simulink library "lut_ram_vhdl"  (R2013b)
settings: Solver=ode45  StartTime=0.0  StopTime=10.0  RelTol=1e-3
libraries: xbsIndex_r4 x27
settings Model: Creator=eyonfen  LastModifiedBy=Administrator

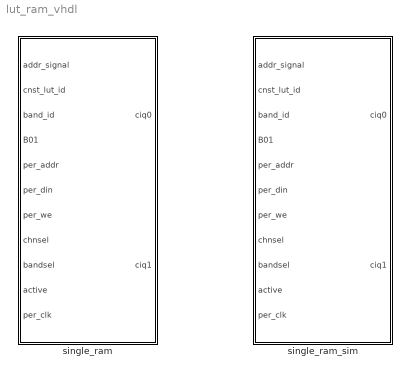
== system lut_ram_vhdl ==
  single_ram : Subsystem
  single_ram_sim : Subsystem

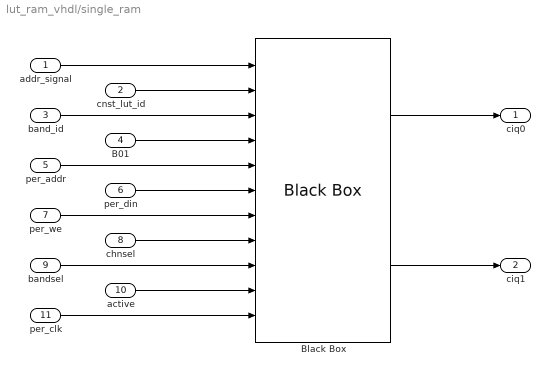
== system lut_ram_vhdl/single_ram ==
  addr_signal : Inport
  cnst_lut_id : Inport  Port=2
  band_id : Inport  Port=3
  B01 : Inport  Port=4
  per_addr : Inport  Port=5
  per_din : Inport  Port=6
  per_we : Inport  Port=7
  chnsel : Inport  Port=8
  bandsel : Inport  Port=9
  active : Inport  Port=10
  per_clk : Inport  Port=11
  Black Box : xbsIndex_r4/Black Box  init_code=dim2lut_config  sim_method=Inactive  verbose=off  block_type=blackbox2
  ciq0 : Outport
  ciq1 : Outport  Port=2
  wires:
  Black Box/1 -> ciq0/1
  Black Box/2 -> ciq1/1
  addr_signal/1 -> Black Box/1
  cnst_lut_id/1 -> Black Box/2
  band_id/1 -> Black Box/3
  B01/1 -> Black Box/4
  per_addr/1 -> Black Box/5
  per_din/1 -> Black Box/6
  per_we/1 -> Black Box/7
  chnsel/1 -> Black Box/8
  bandsel/1 -> Black Box/9
  active/1 -> Black Box/10
  per_clk/1 -> Black Box/11

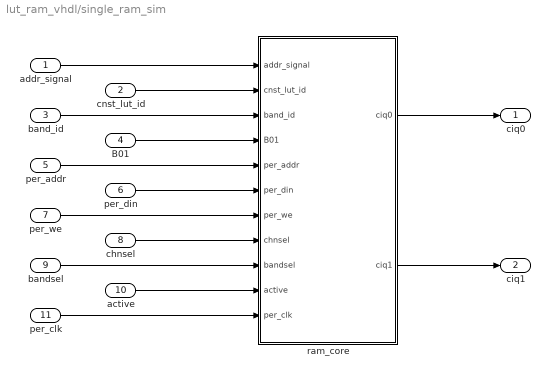
== system lut_ram_vhdl/single_ram_sim ==
  addr_signal : Inport
  cnst_lut_id : Inport  Port=2
  band_id : Inport  Port=3
  B01 : Inport  Port=4
  per_addr : Inport  Port=5
  per_din : Inport  Port=6
  per_we : Inport  Port=7
  chnsel : Inport  Port=8
  bandsel : Inport  Port=9
  active : Inport  Port=10
  per_clk : Inport  Port=11
  ram_core : Subsystem
  ciq0 : Outport
  ciq1 : Outport  Port=2
  wires:
  ram_core/1(ciq0) -> ciq0/1
  ram_core/2(ciq1) -> ciq1/1
  addr_signal/1 -> ram_core/1(addr_signal)
  cnst_lut_id/1 -> ram_core/2(cnst_lut_id)
  band_id/1 -> ram_core/3(band_id)
  B01/1 -> ram_core/4(B01)
  per_addr/1 -> ram_core/5(per_addr)
  per_din/1 -> ram_core/6(per_din)
  per_we/1 -> ram_core/7(per_we)
  chnsel/1 -> ram_core/8(chnsel)
  bandsel/1 -> ram_core/9(bandsel)
  active/1 -> ram_core/10(active)
  per_clk/1 -> ram_core/11(per_clk)

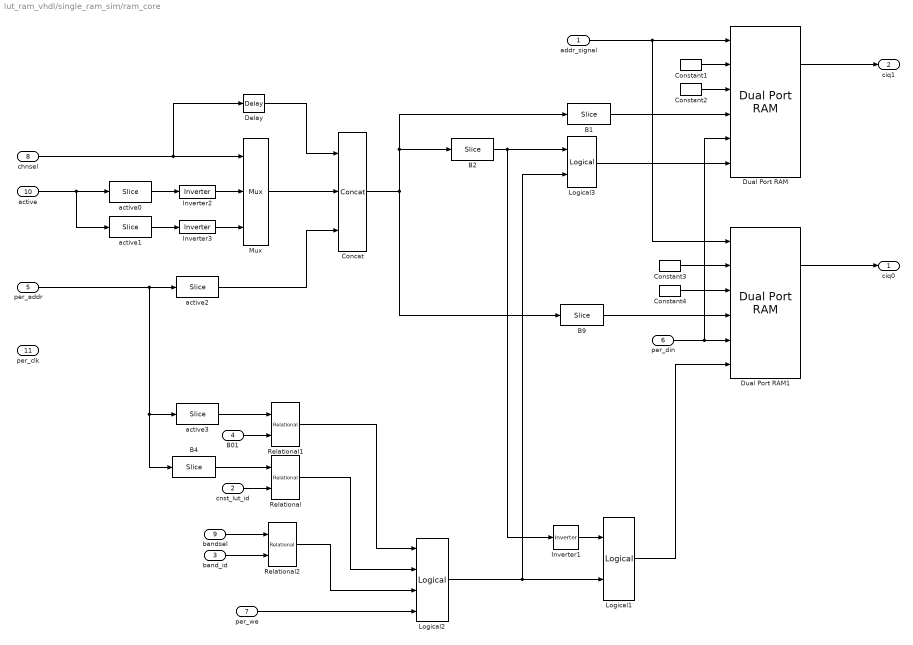
== system lut_ram_vhdl/single_ram_sim/ram_core ==
  addr_signal : Inport
  cnst_lut_id : Inport  Port=2
  band_id : Inport  Port=3
  B01 : Inport  Port=4
  per_addr : Inport  Port=5
  per_din : Inport  Port=6
  per_we : Inport  Port=7
  chnsel : Inport  Port=8
  bandsel : Inport  Port=9
  active : Inport  Port=10
  per_clk : Inport  Port=11
  B1 : xbsIndex_r4/Slice  nbits=9  boolean_output=off  mode=Lower Bit Location + Width  bit1=0  base1=MSB of Input  bit0=1  base0=LSB of Input  dbl_ovrd=off  block_type=slice
  B2 : xbsIndex_r4/Slice  nbits=1  boolean_output=on  mode=Lower Bit Location + Width  bit1=0  base1=MSB of Input  bit0=0  base0=LSB of Input  dbl_ovrd=off  block_type=slice
  B4 : xbsIndex_r4/Slice  nbits=4  boolean_output=off  mode=Lower Bit Location + Width  bit1=0  base1=MSB of Input  bit0=11  base0=LSB of Input  dbl_ovrd=off  block_type=slice
  B9 : xbsIndex_r4/Slice  nbits=9  boolean_output=off  mode=Lower Bit Location + Width  bit1=0  base1=MSB of Input  bit0=1  base0=LSB of Input  dbl_ovrd=off  block_type=slice
  Concat : xbsIndex_r4/Concat  num_inputs=3  dbl_ovrd=off  block_type=concat
  Constant1 : xbsIndex_r4/Constant  const=0  gui_display_data_type=Fixed-point  arith_type=Unsigned  n_bits=32  bin_pt=0  preci_type=Single  exp_width=8  frac_width=24  explicit_period=off  period=1  equ=P=C  opselect=C  inp2=PCIN>>17  opr=+  inp1=P  carry=CIN  dbl_ovrd=off  block_type=constant
  Constant2 : xbsIndex_r4/Constant  const=0  gui_display_data_type=Boolean  arith_type=Boolean  n_bits=16  bin_pt=14  preci_type=Single  exp_width=8  frac_width=24  explicit_period=off  period=1  equ=P=C  opselect=C  inp2=PCIN>>17  opr=+  inp1=P  carry=CIN  dbl_ovrd=off  block_type=constant
  Constant3 : xbsIndex_r4/Constant  const=0  gui_display_data_type=Fixed-point  arith_type=Unsigned  n_bits=32  bin_pt=0  preci_type=Single  exp_width=8  frac_width=24  explicit_period=off  period=1  equ=P=C  opselect=C  inp2=PCIN>>17  opr=+  inp1=P  carry=CIN  dbl_ovrd=off  block_type=constant
  Constant4 : xbsIndex_r4/Constant  const=0  gui_display_data_type=Boolean  arith_type=Boolean  n_bits=16  bin_pt=14  preci_type=Single  exp_width=8  frac_width=24  explicit_period=off  period=1  equ=P=C  opselect=C  inp2=PCIN>>17  opr=+  inp1=P  carry=CIN  dbl_ovrd=off  block_type=constant
  Delay : xbsIndex_r4/Delay  rst=off  infoeditControl=Selection of Reset will increase slice count due to use of real FFs and instead of SRLs  en=off  latency=1  reg_retiming=off  dbl_ovrd=off  block_type=delay
      settings: infoedit=Hardware notes: A delay line is a chain, each link of which is an SRL16 or SRL32 followed by a flip-flop.
  Dual Port RAM : xbsIndex_r4/Dual Port RAM  depth=512  initVector=0  distributed_mem=Block RAM  init_a=0  init_b=0  rst_a=off  rst_b=off  en_a=off  en_b=off  latency=2  write_mode_A=No Read On Write  write_mode_B=No Read On Write  optimize=Speed  dbl_ovrd=off  block_type=dpram
  Dual Port RAM1 : xbsIndex_r4/Dual Port RAM  depth=512  initVector=0  distributed_mem=Block RAM  init_a=0  init_b=0  rst_a=off  rst_b=off  en_a=off  en_b=off  latency=2  write_mode_A=No Read On Write  write_mode_B=No Read On Write  optimize=Speed  dbl_ovrd=off  block_type=dpram
  Inverter1 : xbsIndex_r4/Inverter  en=off  latency=0  dbl_ovrd=off  block_type=inv
  Inverter2 : xbsIndex_r4/Inverter  en=off  latency=0  dbl_ovrd=off  block_type=inv
  Inverter3 : xbsIndex_r4/Inverter  en=off  latency=0  dbl_ovrd=off  block_type=inv
  Logical1 : xbsIndex_r4/Logical  logical_function=AND  inputs=2  en=off  latency=0  precision=Full  arith_type=Unsigned  n_bits=16  bin_pt=0  align_bp=on  dbl_ovrd=off  block_type=logical
  Logical2 : xbsIndex_r4/Logical  logical_function=AND  inputs=4  en=off  latency=0  precision=Full  arith_type=Unsigned  n_bits=16  bin_pt=0  align_bp=on  dbl_ovrd=off  block_type=logical
  Logical3 : xbsIndex_r4/Logical  logical_function=AND  inputs=2  en=off  latency=0  precision=Full  arith_type=Unsigned  n_bits=16  bin_pt=0  align_bp=on  dbl_ovrd=off  block_type=logical
  Mux : xbsIndex_r4/Mux  inputs=2  en=off  latency=1  precision=Full  arith_type=Unsigned  n_bits=16  bin_pt=14  quantization=Truncate  overflow=Wrap  dbl_ovrd=off  block_type=mux
  Relational : xbsIndex_r4/Relational  mode=a=b  op_type=Bool  en=off  latency=0  dbl_ovrd=off  block_type=relational
  Relational1 : xbsIndex_r4/Relational  mode=a=b  op_type=Bool  en=off  latency=0  dbl_ovrd=off  block_type=relational
  Relational2 : xbsIndex_r4/Relational  mode=a=b  op_type=Bool  en=off  latency=0  dbl_ovrd=off  block_type=relational
  active0 : xbsIndex_r4/Slice  nbits=1  boolean_output=off  mode=Lower Bit Location + Width  bit1=0  base1=MSB of Input  bit0=0  base0=LSB of Input  dbl_ovrd=off  block_type=slice
  active1 : xbsIndex_r4/Slice  nbits=1  boolean_output=off  mode=Lower Bit Location + Width  bit1=0  base1=MSB of Input  bit0=1  base0=LSB of Input  dbl_ovrd=off  block_type=slice
  active2 : xbsIndex_r4/Slice  nbits=8  boolean_output=off  mode=Lower Bit Location + Width  bit1=0  base1=MSB of Input  bit0=0  base0=LSB of Input  dbl_ovrd=off  block_type=slice
  active3 : xbsIndex_r4/Slice  nbits=1  boolean_output=off  mode=Lower Bit Location + Width  bit1=0  base1=MSB of Input  bit0=8  base0=LSB of Input  dbl_ovrd=off  block_type=slice
  ciq0 : Outport
  ciq1 : Outport  Port=2
  wires:
  Dual Port RAM/1 -> ciq1/1
  Dual Port RAM1/1 -> ciq0/1
  per_din/1 -> Dual Port RAM1/5, Dual Port RAM/5
  Relational1/1 -> Logical2/1
  Relational2/1 -> Logical2/3
  band_id/1 -> Relational2/2
  bandsel/1 -> Relational2/1
  B01/1 -> Relational1/2
  active3/1 -> Relational1/1
  Logical3/1 -> Dual Port RAM/6
  B2/1 -> Logical3/1, Inverter1/1
  Logical2/1 -> Logical1/2, Logical3/2
  Logical1/1 -> Dual Port RAM1/6
  Inverter1/1 -> Logical1/1
  B1/1 -> Dual Port RAM/4
  B9/1 -> Dual Port RAM1/4
  Concat/1 -> B9/1, B1/1, B2/1
  per_we/1 -> Logical2/4
  Relational/1 -> Logical2/2
  cnst_lut_id/1 -> Relational/2
  B4/1 -> Relational/1
  active2/1 -> Concat/3
  per_addr/1 -> active2/1, B4/1, active3/1
  Mux/1 -> Concat/2
  Delay/1 -> Concat/1
  chnsel/1 -> Mux/1, Delay/1
  active1/1 -> Inverter3/1
  active0/1 -> Inverter2/1
  Inverter2/1 -> Mux/2
  Inverter3/1 -> Mux/3
  active/1 -> active0/1, active1/1
  Constant4/1 -> Dual Port RAM1/3
  Constant3/1 -> Dual Port RAM1/2
  Constant2/1 -> Dual Port RAM/3
  Constant1/1 -> Dual Port RAM/2
  addr_signal/1 -> Dual Port RAM/1, Dual Port RAM1/1
